simulink model "s9dot2_4while"  (R2023b)
settings: Solver=FixedStepAuto  StartTime=0.0  StopTime=120  FixedStep=1  RelTol=1e-3
libraries: simulink x1
settings Model: Creator=lxj  LastModifiedBy=lxj

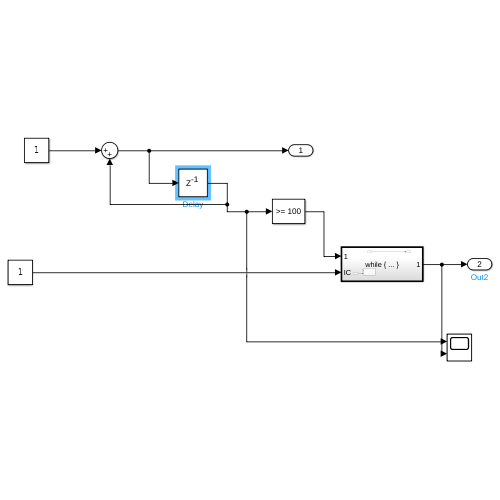
[thumbnail: Simulink's stored preview of the top-level diagram]
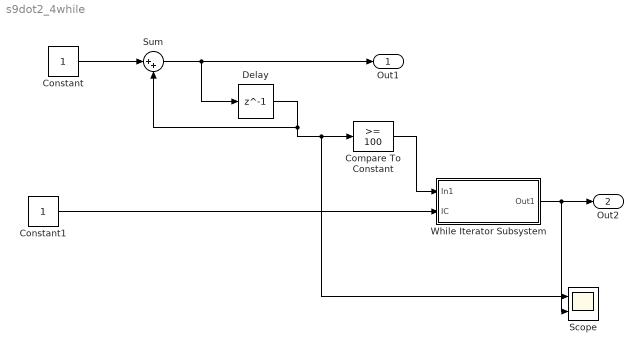
== system s9dot2_4while ==
  Compare To Constant : simulink/Logic and Bit Operations/Compare To Constant  relop=>=  const=100  OutDataTypeStr=boolean
  Constant : Constant
  Constant1 : Constant
  Delay : Delay  DelayLength=1  InitialCondition=0
  Scope : Scope  NumInputPorts=2
  Sum : Sum  Inputs=|++
  While Iterator Subsystem : Subsystem  TreatAsAtomicUnit=on
  Out1 : Outport
  Out2 : Outport  Port=2
  wires:
  Constant/1 -> Sum/1
  Sum/1 -> Out1/1, Delay/1
  Delay/1 -> Scope/1, Compare To Constant/1, Sum/2
  While Iterator Subsystem/1(Out1) -> Scope/2, Out2/1
  Compare To Constant/1 -> While Iterator Subsystem/1(In1)
  Constant1/1 -> While Iterator Subsystem/2(IC)

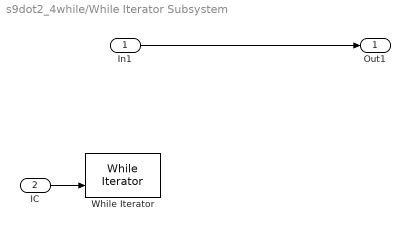
== system s9dot2_4while/While Iterator Subsystem ==
  In1 : Inport
  IC : Inport  Port=2
  While Iterator : WhileIterator
  Out1 : Outport
  wires:
  IC/1 -> While Iterator/2
  In1/1 -> Out1/1
